simulink model "micro_instruction"  (R2020a)
settings: Solver=VariableStepAuto  StartTime=0.0  StopTime=inf  RelTol=1e-3
libraries: simulink_extras x1, hdlsllib x1
settings Model: EnablePacing=on  PacingRate=0.500000  Creator=F1  LastModifiedBy=F1

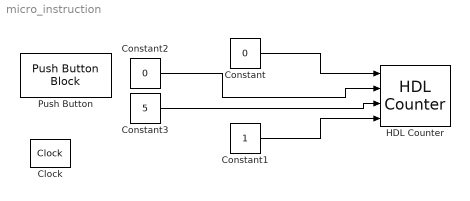
== system micro_instruction ==
  Clock : simulink_extras/Flip Flops/Clock  period=2
  Constant : Constant  Value=0  OutDataTypeStr=boolean
  Constant1 : Constant  OutDataTypeStr=boolean
  Constant2 : Constant  Value=0  OutDataTypeStr=boolean
  Constant3 : Constant  Value=5  OutDataTypeStr=uint8
  HDL Counter : hdlsllib/Sources/HDL Counter  CountType=Count limited  CountInit=0  CountStep=1  CountMax=7  CountFromType=Initial value  CountFrom=0  CountResetPort=on  CountLoadPort=on  CountEnbPort=on  CountDirPort=off  CountDataType=Unsigned  CountWordLen=8  CountFracLen=0  CountSampTime=1
  Push Button : PushButtonBlock
  wires:
  Constant1/1 -> HDL Counter/4
  Constant/1 -> HDL Counter/1
  Constant2/1 -> HDL Counter/2
  Constant3/1 -> HDL Counter/3
